simulink model "GuiamentoControle"  (R2024a)
settings: Solver=FixedStepAuto  StartTime=0.0  StopTime=C.Tfim  FixedStep=0.01  MaxStep=0.001  RelTol=1e-3
values from neighbouring files (symbols this model uses):
  C = CondLanc6DOF    [RunGuiamentoDiag.m]    (also in RunGuiamentoFull.m; RunGuiamentoPlots.m; VooUnico6DOF.m)
  cte_grav = 9.8    [CondLanc6DOF.m]    (also in DadosControle.m; DadosMissil.m; Envelope6DOF.m; RunGuiamentoDiag.m)
  D = DadosControle(D)    [Envelope6DOF.m]    (also in ProjContAlt.m = DadosCGInercia(D); ProjRLocus.m = DadosCGInercia(D); RunGuiamentoDiag.m; RunGuiamentoFull.m)
  R2D = 180/pi    (= 57.2957795131)    [DadosControle.m]    (also in Envelope6DOF.m; RunGuiamentoDiag.m; RunGuiamentoFull.m; RunGuiamentoPlots.m)
  T_acel_k_ext = [0.103333333333 0.121666666667 0.126666666667 0.116666666667 0.143333333333 0.196666666667 0.103333333333 0.121666666667 0.126666666667 0.116666666667 0.143333333333 0.193333333333 ... (36 elements, 6x2x3)]    [autopiloto.mat]    (also in autopiloto_antiship.mat = [0.00333333333333 0.00333333333333 0.00333333333333 0.006666)
  T_acel_k_int = [0.788 0.796 0.789 0.757 0.742 0.695 0.792 0.8 0.793 0.761 0.746 0.699 ... (36 elements, 6x2x3)]    [autopiloto.mat]    (also in autopiloto_antiship.mat = [0.786666666667 1.01333333333 1.14666666667 1.18666666667 1.)
  T_at_k_ext = zeros(length(x_CG),length(altitude),length(Mach))    [ProjRLocus.m]    (also in autopiloto.mat = [5.525 6.1 7.1625 8.4375 9.9 12.1875 5.4875 6.0625 7.1125 8.; autopiloto_antiship.mat = [9.33333333333 13.3333333333 18.6666666667 24 34.6666666667 )
  T_at_k_int = zeros(length(x_CG),length(altitude),length(Mach))    [ProjRLocus.m]    (also in autopiloto.mat = [0.788 0.796 0.789 0.757 0.742 0.695 0.792 0.8 0.793 0.761 0; autopiloto_antiship.mat = [0.786666666667 1.01333333333 1.14666666667 1.18666666667 1.)
  vet_altitude = altitude    [ProjRLocus.m]    (also in autopiloto.mat = [10 100]; autopiloto_antiship.mat = [10 100])
  vet_Mach = Mach    [ProjRLocus.m]    (also in autopiloto.mat = [0.6 0.75 0.9]; autopiloto_antiship.mat = [0.6 0.75 0.9 1])
  vet_x_CG = x_CG    [ProjRLocus.m]    (also in autopiloto.mat = [-2.56109748385 -2.4846531203 -2.35211691443 -2.20935548439 ; autopiloto_antiship.mat = [-2.98430726841 -2.86504003942 -2.66873079492 -2.47886843287)
undefined symbols (not defined in the file or in its folder): dados, M_CD, M_CM, M_CMQ, M_CN, Newton, Raphson
libraries: simulink x14, aerolibasang x9, shared6dof x5, sharedutil x3, aerolibatmos2 x1, dspmtrx3 x1
(part 2 of 2)

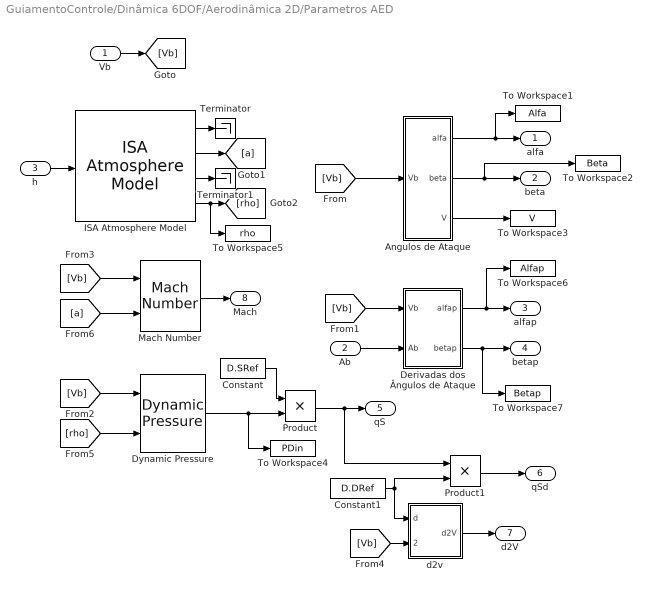
== system GuiamentoControle/Dinâmica 6DOF/Aerodinâmica 2D/Parametros AED ==
  Vb : Inport
  Ab : Inport  Port=2
  h : Inport  Port=3
  Angulos de Ataque : Subsystem
  Constant : Constant  Value=D.SRef
  Constant1 : Constant  Value=D.DRef
  Derivadas dos Ângulos de Ataque : Subsystem
  Dynamic Pressure : aerolibasang/Dynamic Pressure
  ISA Atmosphere Model : aerolibatmos2/ISA Atmosphere Model  custom=off  g=9.80665  gamma=1.4  R=287.0531  L=0.0065  h_trop=11000  h_strat=20000  rho0=1.225  P0=101325  T0=288.15  h0=0
      settings: SourceProductName=Aerospace Blockset
  Mach Number : aerolibasang/Mach Number
      settings: SourceProductName=Aerospace Blockset
  Product : Product
  Product1 : Product
  Terminator : Terminator
  Terminator1 : Terminator
  To Workspace1 : ToWorkspace  VariableName=Alfa  SaveFormat=Timeseries  SampleTime=-1
  To Workspace2 : ToWorkspace  VariableName=Beta  SaveFormat=Timeseries  SampleTime=-1
  To Workspace3 : ToWorkspace  VariableName=V  SaveFormat=Timeseries  SampleTime=-1
  To Workspace4 : ToWorkspace  VariableName=PDin  SaveFormat=Timeseries  SampleTime=-1
  To Workspace5 : ToWorkspace  VariableName=rho  SaveFormat=Timeseries  SampleTime=-1
  To Workspace6 : ToWorkspace  VariableName=Alfap  SaveFormat=Timeseries  SampleTime=-1
  To Workspace7 : ToWorkspace  VariableName=Betap  SaveFormat=Timeseries  SampleTime=-1
  d2v : Subsystem
  alfa : Outport  VectorParamsAs1DForOutWhenUnconnected=off
  beta : Outport  Port=2  VectorParamsAs1DForOutWhenUnconnected=off
  alfap : Outport  Port=3  VectorParamsAs1DForOutWhenUnconnected=off
  betap : Outport  Port=4  VectorParamsAs1DForOutWhenUnconnected=off
  qS : Outport  Port=5  VectorParamsAs1DForOutWhenUnconnected=off
  qSd : Outport  Port=6  VectorParamsAs1DForOutWhenUnconnected=off
  d2V : Outport  Port=7  VectorParamsAs1DForOutWhenUnconnected=off
  Mach : Outport  Port=8  VectorParamsAs1DForOutWhenUnconnected=off
  wires:
  Derivadas dos Ângulos de Ataque/2(betap) -> To Workspace7/1, betap/1
  Derivadas dos Ângulos de Ataque/1(alfap) -> To Workspace6/1, alfap/1
  h/1 -> ISA Atmosphere Model/1
  Constant/1 -> Product/1
  Dynamic Pressure/1 -> To Workspace4/1, Product/2
  ISA Atmosphere Model/4 -> To Workspace5/1, [rho]
  Constant1/1 -> Product1/2, d2v/1(d)
  Product1/1 -> qSd/1
  d2v/1(d2V) -> d2V/1
  Product/1 -> Product1/1, qS/1
  Angulos de Ataque/3(V) -> To Workspace3/1
  Angulos de Ataque/1(alfa) -> To Workspace1/1, alfa/1
  Angulos de Ataque/2(beta) -> beta/1, To Workspace2/1
  Mach Number/1 -> Mach/1
  Vb/1 -> [Vb]
  [Vb] -> Angulos de Ataque/1(Vb)
  [Vb] -> Derivadas dos Ângulos de Ataque/1(Vb)
  [Vb] -> Dynamic Pressure/1
  [Vb] -> Mach Number/1
  [Vb] -> d2v/2(Velocity)
  [rho] -> Dynamic Pressure/2
  [a] -> Mach Number/2
  ISA Atmosphere Model/2 -> [a]
  ISA Atmosphere Model/1 -> Terminator/1
  ISA Atmosphere Model/3 -> Terminator1/1
  Ab/1 -> Derivadas dos Ângulos de Ataque/2(Ab)

== system GuiamentoControle/Dinâmica 6DOF/Aerodinâmica 2D/Subsystem ==
  dltz : Inport
  "Mach " : Inport  Port=2
  alfa : Inport  Port=3
  qS : Inport  Port=4
  Gain1 : Gain  Gain=R2D
  Gain2 : Gain  Gain=R2D
  Gain3 : Gain  Gain=-1
  Product2 : Product
  n-D Lookup Table : Lookup_n-D  NumberOfTableDimensions=3  BreakpointsForDimension1=dados.delta  BreakpointsForDimension2=dados.mach  BreakpointsForDimension3=dados.alpha  Table=M_CN  ExtrapMethod=Clip  InternalRulePriority=Speed  RndMeth=Simplest
      settings: InputPortMap=u0,u1,u2
  Fz : Outport  VectorParamsAs1DForOutWhenUnconnected=off
  wires:
  "Mach "/1 -> n-D Lookup Table/2
  dltz/1 -> Gain2/1
  alfa/1 -> Gain1/1
  Product2/1 -> Gain3/1
  n-D Lookup Table/1 -> Product2/1
  qS/1 -> Product2/2
  Gain2/1 -> n-D Lookup Table/1
  Gain1/1 -> n-D Lookup Table/3
  Gain3/1 -> Fz/1

== system GuiamentoControle/Dinâmica 6DOF/Aerodinâmica 2D/Subsystem1 ==
  "dlty " : Inport
  Mach : Inport  Port=2
  beta : Inport  Port=3
  qS : Inport  Port=4
  Gain2 : Gain  Gain=-R2D
  Gain3 : Gain  Gain=R2D
  Product1 : Product
  n-D Lookup Table : Lookup_n-D  NumberOfTableDimensions=3  BreakpointsForDimension1=dados.delta  BreakpointsForDimension2=dados.mach  BreakpointsForDimension3=dados.alpha  Table=M_CN  ExtrapMethod=Clip  InternalRulePriority=Speed  RndMeth=Simplest
      settings: InputPortMap=u0,u1,u2
  Fy : Outport  VectorParamsAs1DForOutWhenUnconnected=off
  wires:
  n-D Lookup Table/1 -> Product1/1
  beta/1 -> Gain2/1
  "dlty "/1 -> Gain3/1
  Mach/1 -> n-D Lookup Table/2
  qS/1 -> Product1/2
  Gain3/1 -> n-D Lookup Table/1
  Gain2/1 -> n-D Lookup Table/3
  Product1/1 -> Fy/1

== system GuiamentoControle/Dinâmica 6DOF/Aerodinâmica 2D/Subsystem2 ==
  alfa : Inport
  qS : Inport  Port=2
  dltz : Inport  Port=3
  "Mach " : Inport  Port=4
  beta : Inport  Port=5
  dlty : Inport  Port=6
  Add : Sum  Inputs=++-
  Constant : Constant  Value=0
  Gain : Gain  Gain=-1
  Gain{1..4} (4 alike) : Gain  Gain=R2D
  Gain5 : Gain
  Gain6 : Gain
  Gain7 : Gain
  Product : Product
  n-D Lookup Table : Lookup_n-D  NumberOfTableDimensions=3  BreakpointsForDimension1=dados.delta  BreakpointsForDimension2=dados.mach  BreakpointsForDimension3=dados.alpha  Table=M_CD  ExtrapMethod=Clip  InternalRulePriority=Speed  RndMeth=Simplest
      settings: InputPortMap=u0,u1,u2
  n-D Lookup Table1 : Lookup_n-D  NumberOfTableDimensions=3  BreakpointsForDimension1=dados.delta  BreakpointsForDimension2=dados.mach  BreakpointsForDimension3=dados.alpha  Table=M_CD  ExtrapMethod=Clip  InternalRulePriority=Speed  RndMeth=Simplest
      settings: InputPortMap=u0,u1,u2
  n-D Lookup Table2 : Lookup_n-D  NumberOfTableDimensions=3  BreakpointsForDimension1=dados.delta  BreakpointsForDimension2=dados.mach  BreakpointsForDimension3=dados.alpha  Table=M_CD  ExtrapMethod=Clip  InternalRulePriority=Speed  RndMeth=Simplest
      settings: InputPortMap=u0,u1,u2
  Fx : Outport  VectorParamsAs1DForOutWhenUnconnected=off
  wires:
  qS/1 -> Product/2
  Gain3/1 -> n-D Lookup Table/1
  Gain2/1 -> n-D Lookup Table/3
  Product/1 -> Fx/1
  Gain1/1 -> n-D Lookup Table1/3
  Gain4/1 -> n-D Lookup Table1/1
  Constant/1 -> n-D Lookup Table2/3, n-D Lookup Table2/1
  n-D Lookup Table2/1 -> Gain5/1
  "Mach "/1 -> n-D Lookup Table2/2, n-D Lookup Table1/2, n-D Lookup Table/2
  n-D Lookup Table/1 -> Gain7/1
  n-D Lookup Table1/1 -> Gain6/1
  Add/1 -> Gain/1
  Gain/1 -> Product/1
  dltz/1 -> Gain3/1
  alfa/1 -> Gain2/1
  dlty/1 -> Gain4/1
  beta/1 -> Gain1/1
  Gain5/1 -> Add/3
  Gain6/1 -> Add/2
  Gain7/1 -> Add/1

== system GuiamentoControle/Dinâmica 6DOF/Aerodinâmica 2D/Subsystem3 ==
  dlty : Inport
  Mach : Inport  Port=2
  beta : Inport  Port=3
  qSd : Inport  Port=4
  r : Inport  Port=5
  d2V : Inport  Port=6
  betap : Inport  Port=7
  Add : Sum  Inputs=+++
  Constant : Constant  Value=D.Cmap
  Gain1 : Gain  Gain=-R2D
  Gain2 : Gain  Gain=R2D
  Product1 : Product  Inputs=3
  Product4 : Product  Inputs=3
  Product6 : Product
  n-D Lookup Table : Lookup_n-D  NumberOfTableDimensions=3  BreakpointsForDimension1=dados.delta  BreakpointsForDimension2=dados.mach  BreakpointsForDimension3=dados.alpha  Table=M_CM  ExtrapMethod=Clip  InternalRulePriority=Speed  RndMeth=Simplest
      settings: InputPortMap=u0,u1,u2
  n-D Lookup Table1 : Lookup_n-D  NumberOfTableDimensions=3  BreakpointsForDimension1=dados.delta  BreakpointsForDimension2=dados.mach  BreakpointsForDimension3=dados.alpha  Table=M_CMQ  ExtrapMethod=Clip  InternalRulePriority=Speed  RndMeth=Simplest
      settings: InputPortMap=u0,u1,u2
  N : Outport  VectorParamsAs1DForOutWhenUnconnected=off
  wires:
  d2V/1 -> Product1/1, Product4/3
  Product6/1 -> N/1
  Add/1 -> Product6/1
  qSd/1 -> Product6/2
  r/1 -> Product4/2
  dlty/1 -> Gain2/1
  Mach/1 -> n-D Lookup Table1/2, n-D Lookup Table/2
  beta/1 -> Gain1/1
  Product4/1 -> Add/2
  Gain2/1 -> n-D Lookup Table/1, n-D Lookup Table1/1
  Gain1/1 -> n-D Lookup Table/3, n-D Lookup Table1/3
  n-D Lookup Table/1 -> Add/1
  n-D Lookup Table1/1 -> Product4/1
  Constant/1 -> Product1/3
  Product1/1 -> Add/3
  betap/1 -> Product1/2

== system GuiamentoControle/Dinâmica 6DOF/Aerodinâmica 2D/Subsystem4 ==
  dltz : Inport
  Mach : Inport  Port=2
  alfa : Inport  Port=3
  qSd : Inport  Port=4
  q : Inport  Port=5
  d2V : Inport  Port=6
  alfap : Inport  Port=7
  Add : Sum  Inputs=+++
  Constant : Constant  Value=D.Cmap
  Gain1 : Gain  Gain=R2D
  Gain2 : Gain  Gain=R2D
  Product1 : Product  Inputs=3
  Product4 : Product  Inputs=3
  Product6 : Product
  n-D Lookup Table : Lookup_n-D  NumberOfTableDimensions=3  BreakpointsForDimension1=dados.delta  BreakpointsForDimension2=dados.mach  BreakpointsForDimension3=dados.alpha  Table=M_CM  ExtrapMethod=Clip  InternalRulePriority=Speed  RndMeth=Simplest
      settings: InputPortMap=u0,u1,u2
  n-D Lookup Table1 : Lookup_n-D  NumberOfTableDimensions=3  BreakpointsForDimension1=dados.delta  BreakpointsForDimension2=dados.mach  BreakpointsForDimension3=dados.alpha  Table=M_CMQ  ExtrapMethod=Clip  InternalRulePriority=Speed  RndMeth=Simplest
      settings: InputPortMap=u0,u1,u2
  M : Outport  VectorParamsAs1DForOutWhenUnconnected=off
  wires:
  d2V/1 -> Product1/1, Product4/3
  Product6/1 -> M/1
  Add/1 -> Product6/1
  qSd/1 -> Product6/2
  q/1 -> Product4/2
  dltz/1 -> Gain2/1
  alfa/1 -> Gain1/1
  Product4/1 -> Add/2
  Gain2/1 -> n-D Lookup Table1/1, n-D Lookup Table/1
  Gain1/1 -> n-D Lookup Table/3, n-D Lookup Table1/3
  n-D Lookup Table/1 -> Add/1
  n-D Lookup Table1/1 -> Product4/1
  Mach/1 -> n-D Lookup Table/2, n-D Lookup Table1/2
  alfap/1 -> Product1/2
  Product1/1 -> Add/3
  Constant/1 -> Product1/3

== system GuiamentoControle/Guiamento e Controle/Guiamento Terminal/Compensação Gravidade ==
  DCM : Inport
  Constant3 : Constant  Value=0
  Constant4 : Constant  Value=0
  Constant5 : Constant  Value=-cte_grav
  Mux : Mux  Inputs=3
  "transform to Inertial axes " : shared6dof/6DOF (Euler Angles)/transform to Inertial axes   SystemSampleTime=-1
      settings: SourceProductName=Aerospace Blockset
  g_b : Outport  VectorParamsAs1DForOutWhenUnconnected=off
  wires:
  Constant3/1 -> Mux/1
  DCM/1 -> "transform to Inertial axes "/2
  Mux/1 -> "transform to Inertial axes "/1
  "transform to Inertial axes "/1 -> g_b/1
  Constant5/1 -> Mux/3
  Constant4/1 -> Mux/2

== system GuiamentoControle/Dinâmica 6DOF/Aerodinâmica 2D/Parametros AED/Angulos de Ataque ==
  Vb : Inport
  Airspeed : Sqrt  AlgorithmType=Newton-Raphson
  Demux1 : Demux  Outputs=3
      settings: DisplayOption=none
  Incidence : Trigonometry  Operator=atan2
  Incidence1 : Trigonometry  Operator=atan2
  dot : aerolibasang/Incidence, Sideslip, & Airspeed/dot  SystemSampleTime=-1
      settings: SourceProductName=Aerospace Blockset
  alfa : Outport  VectorParamsAs1DForOutWhenUnconnected=off
  beta : Outport  Port=2  VectorParamsAs1DForOutWhenUnconnected=off
  V : Outport  Port=3  VectorParamsAs1DForOutWhenUnconnected=off
  wires:
  Demux1/3 -> Incidence/1
  Incidence/1 -> alfa/1
  Vb/1 -> Demux1/1, dot/1
  Demux1/2 -> Incidence1/1
  dot/1 -> Airspeed/1
  Airspeed/1 -> V/1
  Incidence1/1 -> beta/1
  Demux1/1 -> Incidence/2, Incidence1/2

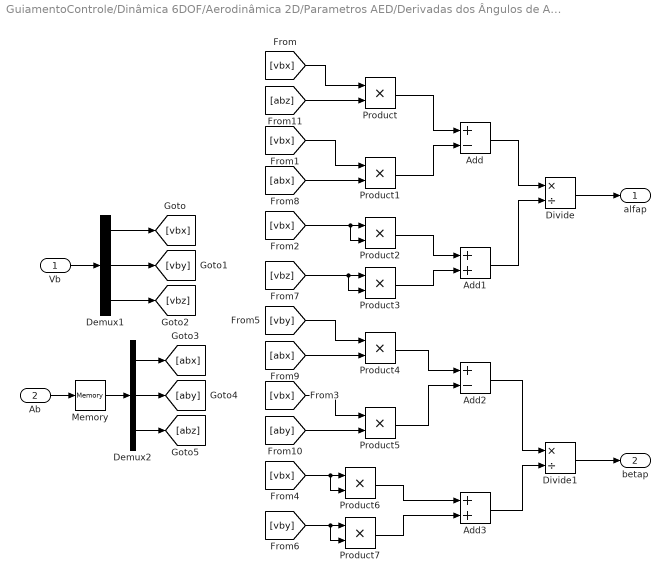
== system GuiamentoControle/Dinâmica 6DOF/Aerodinâmica 2D/Parametros AED/Derivadas dos Ângulos de Ataque ==
  Vb : Inport
  Ab : Inport  Port=2
  Add : Sum  Inputs=+-
  Add1 : Sum
  Add2 : Sum  Inputs=+-
  Add3 : Sum
  Demux1 : Demux  Outputs=3
  Demux2 : Demux  Outputs=3
  Divide : Product  Inputs=*/
  Divide1 : Product  Inputs=*/
  Memory : Memory
  Product{,1..7} (8 alike) : Product
  alfap : Outport  VectorParamsAs1DForOutWhenUnconnected=off
  betap : Outport  Port=2  VectorParamsAs1DForOutWhenUnconnected=off
  wires:
  Product/1 -> Add/1
  Product1/1 -> Add/2
  Product2/1 -> Add1/1
  Product3/1 -> Add1/2
  Add/1 -> Divide/1
  Add1/1 -> Divide/2
  Divide/1 -> alfap/1
  Product4/1 -> Add2/1
  Divide1/1 -> betap/1
  Product7/1 -> Add3/2
  Add2/1 -> Divide1/1
  Product6/1 -> Add3/1
  Product5/1 -> Add2/2
  Add3/1 -> Divide1/2
  Vb/1 -> Demux1/1
  Demux1/1 -> [vbx]
  Demux1/2 -> [vby]
  Demux1/3 -> [vbz]
  [vbx] -> Product/1
  [vbx] -> Product1/1
  [vbx] -> Product2/2, Product2/1
  [vbx] -> Product5/1
  [vbx] -> Product6/2, Product6/1
  [vby] -> Product4/1
  [vby] -> Product7/2, Product7/1
  [vbz] -> Product3/2, Product3/1
  Memory/1 -> Demux2/1
  Ab/1 -> Memory/1
  Demux2/1 -> [abx]
  Demux2/2 -> [aby]
  Demux2/3 -> [abz]
  [abx] -> Product1/2
  [abx] -> Product4/2
  [aby] -> Product5/2
  [abz] -> Product/2

== system GuiamentoControle/Dinâmica 6DOF/Aerodinâmica 2D/Parametros AED/d2v ==
  d : Inport
  Velocity : Inport  Port=2
  Divide : Product  Inputs=*/
  d/(2V) : Gain  Gain=1/2  SaturateOnIntegerOverflow=on  OutDataTypeStr=Inherit: Same as input  ParamDataTypeStr=Inherit: Same as input
  dot : aerolibasang/Dynamic Pressure/dot  SystemSampleTime=-1
      settings: SourceProductName=Aerospace Blockset
  vt : Sqrt  AlgorithmType=Newton-Raphson
  d2V : Outport  InitialOutput=0  VectorParamsAs1DForOutWhenUnconnected=off
  wires:
  d/(2V)/1 -> d2V/1
  Velocity/1 -> dot/1
  Divide/1 -> d/(2V)/1
  dot/1 -> vt/1
  d/1 -> Divide/1
  vt/1 -> Divide/2
